simulink model "HANcoder_E407_TTA_CombineModel_Membership_2022a"  (R2023a)
settings: Solver=FixedStepDiscrete  StartTime=0.0  StopTime=1  FixedStep=0.001  RelTol=1e-3
PreLoadFcn:
  | librarySetup
  | eval([bdroot,'_startup']) %Calling [modelName]_startup.m
values from neighbouring files (symbols this model uses):
  ClockOn = Simulink.Parameter    [HANcoder_E407_TTA_Chris_startup.m]    (also in HANcoder_E407_TTA_CombineModel_Membership_2022a_startup.m; HANcoder_E407_TTA_CombineModel_Membership_startup.m; HANcoder_E407_TTA_CombineModel_V2_startup.m; HANcoder_E407_TTA_CombineModel_startup.m)
  controlWidth = Simulink.Parameter    [HANcoder_E407_TTA_CombineModel_Membership_2022a_startup.m]    (also in HANcoder_E407_TTA_CombineModel_Membership_startup.m; HANcoder_E407_TTA_CombineModel_V2_startup.m)
  desiredAngle = Simulink.Parameter    [HANcoder_E407_TTA_CombineModel_Membership_2022a_startup.m]    (also in HANcoder_E407_TTA_CombineModel_Membership_startup.m; HANcoder_E407_TTA_CombineModel_V2_startup.m)
  ErrorBoard1 = Simulink.Parameter    [HANcoder_E407_TTA_CombineModel_Membership_2022a_startup.m]
  ErrorBoard2 = Simulink.Parameter    [HANcoder_E407_TTA_CombineModel_Membership_2022a_startup.m]
  ErrorBoard3 = Simulink.Parameter    [HANcoder_E407_TTA_CombineModel_Membership_2022a_startup.m]
  ErrorBoard4 = Simulink.Parameter    [HANcoder_E407_TTA_CombineModel_Membership_2022a_startup.m]
  ErrorBoard5 = Simulink.Parameter    [HANcoder_E407_TTA_CombineModel_Membership_2022a_startup.m]
  frequency_IRQ = 1000    [HANcoder_E407_TTA_Chris_startup.m]    (also in HANcoder_E407_TTA_CombineModel_Membership_2022a_startup.m; HANcoder_E407_TTA_CombineModel_Membership_startup.m; HANcoder_E407_TTA_CombineModel_V2_startup.m; HANcoder_E407_TTA_CombineModel_startup.m)
  intVal = Simulink.Parameter    [HANcoder_E407_TTA_CombineModel_Membership_2022a_startup.m]    (also in HANcoder_E407_TTA_CombineModel_Membership_startup.m; HANcoder_E407_TTA_CombineModel_V2_startup.m)
  L0b = 1    [HANcoder_E407_KinematicAngleControl_startup.m]    (also in HANcoder_E407_TTA_CombineModel_Membership_2022a_startup.m; HANcoder_E407_TTA_CombineModel_Membership_startup.m; HANcoder_E407_TTA_CombineModel_V2_startup.m; HANcoder_E407_TTA_CombineModel_startup.m)
  L0F = 3    [HANcoder_E407_KinematicAngleControl_startup.m]    (also in HANcoder_E407_TTA_CombineModel_Membership_2022a_startup.m; HANcoder_E407_TTA_CombineModel_Membership_startup.m; HANcoder_E407_TTA_CombineModel_V2_startup.m; HANcoder_E407_TTA_CombineModel_startup.m)
  L1F = 4    [HANcoder_E407_KinematicAngleControl_startup.m]    (also in HANcoder_E407_TTA_CombineModel_Membership_2022a_startup.m; HANcoder_E407_TTA_CombineModel_Membership_startup.m; HANcoder_E407_TTA_CombineModel_V2_startup.m; HANcoder_E407_TTA_CombineModel_startup.m)
  matrixRows = Simulink.Parameter    [HANcoder_E407_TTA_Chris_startup.m]    (also in HANcoder_E407_TTA_CombineModel_Membership_2022a_startup.m; HANcoder_E407_TTA_CombineModel_Membership_startup.m; HANcoder_E407_TTA_CombineModel_V2_startup.m; HANcoder_E407_TTA_CombineModel_startup.m)
  MMBS1_ID = Simulink.Parameter    [HANcoder_E407_TTA_Chris_startup.m]    (also in HANcoder_E407_TTA_CombineModel_Membership_2022a_startup.m; HANcoder_E407_TTA_CombineModel_Membership_startup.m; HANcoder_E407_TTA_CombineModel_V2_startup.m; HANcoder_E407_TTA_CombineModel_startup.m)
  propVal = Simulink.Parameter    [HANcoder_E407_TTA_CombineModel_Membership_2022a_startup.m]    (also in HANcoder_E407_TTA_CombineModel_Membership_startup.m; HANcoder_E407_TTA_CombineModel_V2_startup.m)
  slotTime = Simulink.Parameter    [HANcoder_E407_TTA_Chris_startup.m]    (also in HANcoder_E407_TTA_CombineModel_Membership_2022a_startup.m; HANcoder_E407_TTA_CombineModel_Membership_startup.m; HANcoder_E407_TTA_CombineModel_V2_startup.m; HANcoder_E407_TTA_CombineModel_startup.m)
  SSTM1_ID = Simulink.Parameter    [HANcoder_E407_TTA_Chris_startup.m]    (also in HANcoder_E407_TTA_CombineModel_Membership_2022a_startup.m; HANcoder_E407_TTA_CombineModel_Membership_startup.m; HANcoder_E407_TTA_CombineModel_V2_startup.m; HANcoder_E407_TTA_CombineModel_startup.m)
  SYNC1_ID = Simulink.Parameter    [HANcoder_E407_TTA_Chris_startup.m]    (also in HANcoder_E407_TTA_CombineModel_Membership_2022a_startup.m; HANcoder_E407_TTA_CombineModel_Membership_startup.m; HANcoder_E407_TTA_CombineModel_V2_startup.m; HANcoder_E407_TTA_CombineModel_startup.m)
  TRCK1_ID1 = Simulink.Parameter    [HANcoder_E407_TTA_Chris_startup.m]    (also in HANcoder_E407_TTA_CombineModel_Membership_2022a_startup.m; HANcoder_E407_TTA_CombineModel_Membership_startup.m; HANcoder_E407_TTA_CombineModel_V2_startup.m; HANcoder_E407_TTA_CombineModel_startup.m)
  TRCK1_ID2 = Simulink.Parameter    [HANcoder_E407_TTA_Chris_startup.m]    (also in HANcoder_E407_TTA_CombineModel_Membership_2022a_startup.m; HANcoder_E407_TTA_CombineModel_Membership_startup.m; HANcoder_E407_TTA_CombineModel_V2_startup.m; HANcoder_E407_TTA_CombineModel_startup.m)
  TRCK1_ID3 = Simulink.Parameter    [HANcoder_E407_TTA_Chris_startup.m]    (also in HANcoder_E407_TTA_CombineModel_Membership_2022a_startup.m; HANcoder_E407_TTA_CombineModel_Membership_startup.m; HANcoder_E407_TTA_CombineModel_V2_startup.m; HANcoder_E407_TTA_CombineModel_startup.m)
  TRLS1_ID4 = Simulink.Parameter    [HANcoder_E407_TTA_Chris_startup.m]    (also in HANcoder_E407_TTA_CombineModel_Membership_2022a_startup.m; HANcoder_E407_TTA_CombineModel_Membership_startup.m; HANcoder_E407_TTA_CombineModel_V2_startup.m; HANcoder_E407_TTA_CombineModel_startup.m)
  TRLS1_ID5 = Simulink.Parameter    [HANcoder_E407_TTA_Chris_startup.m]    (also in HANcoder_E407_TTA_CombineModel_Membership_2022a_startup.m; HANcoder_E407_TTA_CombineModel_Membership_startup.m; HANcoder_E407_TTA_CombineModel_V2_startup.m; HANcoder_E407_TTA_CombineModel_startup.m)
undefined symbols (not defined in the file or in its folder): A2, A3, A4, CON2, CON3, CON4, D10, D4, D5
libraries: HANcoder_STM32_Target x23, hdlsllib x12, dspstat3 x2, simulink_extras x2, simulink x1, slpidlib x1, dspswit3 x1
(part 3 of 4)

== system HANcoder_E407_TTA_CombineModel_Membership_2022a/HANcoder STM32 Target - E407-STM32 algorithm/Message selector/SYNC1_TX/CAN send1 ==
  In1 : Inport
  In2 : Inport  Port=2
  In3 : Inport  Port=3
  In4 : Inport  Port=4
  In5 : Inport  Port=5
  In6 : Inport  Port=6
  In7 : Inport  Port=7
  In8 : Inport  Port=8
  In9 : Inport  Port=9
  S-Function : M-S-Function  FunctionName=sfcn_can_send  Parameters=tsamp, canBus, frameType, inputNumber, dataType, byteOrder
  wires:
  In1/1 -> S-Function/1
  In2/1 -> S-Function/2
  In3/1 -> S-Function/3
  In4/1 -> S-Function/4
  In5/1 -> S-Function/5
  In6/1 -> S-Function/6
  In7/1 -> S-Function/7
  In8/1 -> S-Function/8
  In9/1 -> S-Function/9

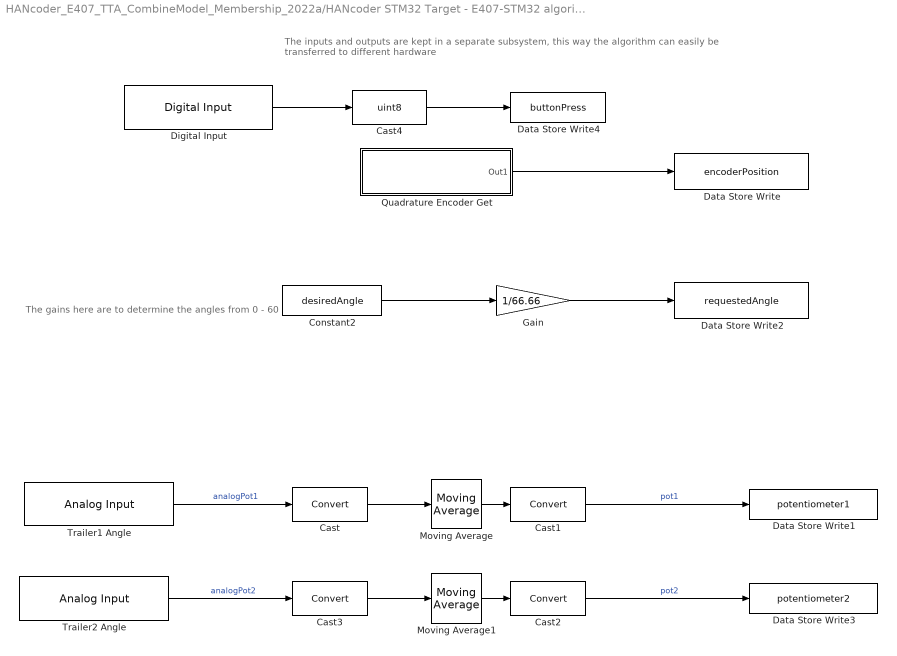
== system HANcoder_E407_TTA_CombineModel_Membership_2022a/HANcoder STM32 Target - E407-STM32 algorithm/Message selector/Slot 5 execution/Inputs ==
  note: The inputs and outputs are kept in a separate subsystem, this way the algorithm can easily be transferred to different hardware
  note: The gains here are to determine the angles from 0 - 60
  Cast{,1..3} (4 alike) : DataTypeConversion  SaturateOnIntegerOverflow=off  RndMeth=Floor
  Cast4 : DataTypeConversion  OutDataTypeStr=uint8  SaturateOnIntegerOverflow=off  RndMeth=Floor
  Constant2 : Constant  Value=desiredAngle
  Data Store Write : DataStoreWrite  DataStoreName=encoderPosition  IndexOptions=Index vector (dialog)  Indices=1  OutputSizes=1
  Data Store Write1 : DataStoreWrite  DataStoreName=potentiometer1  IndexOptions=Index vector (dialog)  Indices=1  OutputSizes=1
  Data Store Write2 : DataStoreWrite  DataStoreName=requestedAngle  IndexOptions=Index vector (dialog)  Indices=1  OutputSizes=1
  Data Store Write3 : DataStoreWrite  DataStoreName=potentiometer2  IndexOptions=Index vector (dialog)  Indices=1  OutputSizes=1
  Data Store Write4 : DataStoreWrite  DataStoreName=buttonPress  IndexOptions=Index vector (dialog)  Indices=1  OutputSizes=1
  Digital Input : HANcoder_STM32_Target/STM32-E407/Digital Inputs/Digital Input  Tag=HANcoder_TARGET_STM32_E407  pinID=WKUP button  config=Pulldown  tsamp=-1
      settings: SourceProductName=HANcoder STM32 Target
  Gain : Gain  Gain=1/66.66  OutDataTypeStr=double  RndMeth=Round
  Moving Average : dspstat3/Moving Average  Method=Sliding window  ForgettingFactorPort=off  SpecifyWindowLength=on  WindowLength=60  OverlapLength=59  AllowArbitraryInputLength=off  ForgettingFactor=0.9  SimulateUsing=Code generation
  Moving Average1 : dspstat3/Moving Average  Method=Sliding window  ForgettingFactorPort=off  SpecifyWindowLength=on  WindowLength=60  OverlapLength=59  AllowArbitraryInputLength=off  ForgettingFactor=0.9  SimulateUsing=Code generation
  Quadrature Encoder Get : Subsystem  Tag=HANcoder_TARGET_STM32_E407  AncestorBlock=HANcoder_STM32_Target/STM32-E407/Timer Inputs/Quadrature Encoder Get  mask(Quadrature Encoder Inputs){moduleID=TIM3: CON4 - D12 & D11 (5V Tolerant), config=Floating, counterReset=off, tsamp=-1}
      mask prompts: moduleID "Quad encoder module"; config "Configuration"; counterReset "Show counter reset input"; tsamp "Sample time"
      mask help:
      | Function
      | ========
      | Reads the counter of the quadrature encoder module.
      |
      | Parameters
      | ==========
      | Quadrature encoder module:
      |   Selects the quadrature encoder module. The channel A and B signals of the
      |   encoder should be connected to the 2 input pins that belong to the module.
      |
      | Configuration:
      |   Determines if the input is floating or is connected to an internal
      |   pull-up or pull-down resistor.
      |
      | Show counter reset input:
      |   Configures if the input port for the counter reset should be shown.
      |
      |
      | Outport
      | ==========
      | 32-bit signed counter. The counter starts at zero and counts up or down
      | depending on the direction of the motor.
      mask init:
      | moduleIDInfoStr = sfcn_quad_encoder_get_mcb(2,moduleID, counterReset, config);
      settings: LibrarySourceBlock=HANcoder_STM32_Target/STM32-E407/Timer Inputs/Quadrature Encoder Get  CopyFcn=sfcn_quad_encoder_get_chk();  MoveFcn=drawLogos
      mask Help: web('sfcn_quad_encoder_get.html');
      mask TypeOptions moduleID: TIM1: CON PE - 12 & 14 (5V Tolerant) | TIM3: CON4 - D12 & D11 (5V Tolerant) | TIM4: CON PD - 15 & 16 (5V Tolerant) | TIM8: UEXT - 3 & 4 (5V Tolerant)
      mask Callback moduleID: sfcn_quad_encoder_get_chk();
      mask TypeOptions config: Floating | Pullup | Pulldown
      mask Display: fprintf('Quad Encoder Get\n%s', moduleIDInfoStr);patch([135 141 141],[8 14 2],[1 0 0]);patch([143 143 149],[14 2 8],[0 0 0.35]);
  Trailer1 Angle : HANcoder_STM32_Target/STM32-E407/Analog Inputs/Analog Input  Tag=HANcoder_TARGET_STM32_E407  pinID=CON2 - A2  tsamp=-1  filtered=off
      settings: SourceProductName=HANcoder STM32 Target
  Trailer2 Angle : HANcoder_STM32_Target/STM32-E407/Analog Inputs/Analog Input  Tag=HANcoder_TARGET_STM32_E407  pinID=CON2 - A3  tsamp=-1  filtered=off
      settings: SourceProductName=HANcoder STM32 Target
  wires:
  Constant2/1 -> Gain/1
  Gain/1 -> Data Store Write2/1
  Quadrature Encoder Get/1(Out1) -> Data Store Write/1
  Trailer1 Angle/1 -> Cast/1  "analogPot1"
  Trailer2 Angle/1 -> Cast3/1  "analogPot2"
  Moving Average/1 -> Cast1/1
  Moving Average1/1 -> Cast2/1
  Cast/1 -> Moving Average/1
  Cast1/1 -> Data Store Write1/1  "pot1"
  Cast2/1 -> Data Store Write3/1  "pot2"
  Cast3/1 -> Moving Average1/1
  Digital Input/1 -> Cast4/1
  Cast4/1 -> Data Store Write4/1

== system HANcoder_E407_TTA_CombineModel_Membership_2022a/HANcoder STM32 Target - E407-STM32 algorithm/Message selector/Slot 5 execution/Outputs ==
  note: The inputs and outputs are kept in a separate subsystem, this way the algorithm can easily be transferred to different hardware
  PWM mospeed : Inport
  CW signal : Inport  Port=2
  CCW signal : Inport  Port=3
  Node : Inport  Port=4
  Data Store Read : DataStoreRead  DataStoreName=Master_ID  IndexOptions=Index vector (dialog)  Indices=1  OutputSizes=1
  Digital Output : HANcoder_STM32_Target/STM32-E407/Digital Outputs/Digital Output  Tag=HANcoder_TARGET_STM32_E407  pinID=CON3 - D4  config=Push pull  tsamp=-1
      settings: SourceProductName=HANcoder STM32 Target
  Digital Output1 : HANcoder_STM32_Target/STM32-E407/Digital Outputs/Digital Output  Tag=HANcoder_TARGET_STM32_E407  pinID=CON3 - D5  config=Push pull  tsamp=-1
      settings: SourceProductName=HANcoder STM32 Target
  Digital Output2 : HANcoder_STM32_Target/STM32-E407/Digital Outputs/Digital Output  Tag=HANcoder_TARGET_STM32_E407  pinID=LED  config=Push pull  tsamp=-1
      settings: SourceProductName=HANcoder STM32 Target
  Equal : RelationalOperator  Operator===  OutDataTypeStr=boolean  RndMeth=Simplest  InputSameDT=off
  PWM Duty Cycle : HANcoder_STM32_Target/STM32-E407/PWM Outputs/PWM Duty Cycle  Tag=HANcoder_TARGET_STM32_E407  pinID=CON2 - A4  tsamp=-1
      settings: SourceProductName=HANcoder STM32 Target
  PWM Init : Subsystem  Tag=HANcoder_TARGET_STM32_E407  AncestorBlock=HANcoder_STM32_Target/STM32-E407/PWM Outputs/PWM Init  mask(Pulse Width Modulation Initialization){moduleID=TIM14: A4 & n/a & n/a & n/a, frequency=10253, alignment=Edge aligned, enableIRQoutput=off, ch1On=on, ch1Pol=Active high, ch1Inv=off, ch2On=on, ch2Pol=Active high, ch2Inv=off, ch3On=off, ch3Pol=Active high, ch3Inv=off, ch4On=off, ch4Pol=Active high, ch4Inv=off}
      mask prompts: moduleID "PWM module"; frequency "Signal frequency [Hz]"; alignment "Signal alignment"; enableIRQoutput "Enable IRQ output"; ch1On "Generate PWM signal on channel 1"; ch1Pol "Select signal polarity"; ch1Inv "Enable inverted signal on additional output pin"; ch2On "Generate PWM signal on channel 2"; ch2Pol "Select signal polarity"; ch2Inv "Enable inverted signal on additional output pin"; ch3On "Generate PWM signal on channel 3"; ch3Pol "Select signal polarity"; ch3Inv "Enable inverted signal on additional output pin"; ch4On "Generate PWM signal on channel 4"; ch4Pol "Select signal polarity"; ch4Inv "Enable inverted signal on additional output pin"
      mask help:
      | Function
      | ========
      | A 'PWM Init' block configures one of the STM32 timer modules for PWM
      | functionality, allowing a PWM signal to be generated on up to 4 timer
      | channels and their associated output pins.
      |
      | Parameters
      | ==========
      | General - PWM module:
      |   Select the PWM module to use. The name in the combo box contains
      |   information about which pins on the target belong to this timer module.
      |   Also the first pin corresponds with the first channel and so on:
      |   TIMx: Ch1 & Ch2 & Ch3...
      |
      | General - Signal frequency:
      |   Determines the signal frequency in Hz. If you click 'Apply' after entering
      |   the desired frequency it will automatically be adjusted to the closest
      |   supported value.
      |
      | General - Signal Aligment:
      |   Determines the aligment of the signal. It can either be edge aligned or
      |   center aligned.
      |
      | General - Enable IRQ output
      |   Controls whether or not the IRQ output is available.
      |
      | Channel x - Generate PWM signal on channel x:
      |   Enable to configure the channel for PWM functionality so that the PWM signal
      |   is outputted on the channel's associated microcontroller pin.
      |
      | Channel x - Signal polarity:
      |   Selects the polarity of the signal.
      |
      | Channel x - Enable inverted signal on additional output pin:
      |   When enabled, a second PWM signal will be generated on an additional
      |   microcontroller pin where the signal is an exact inversion of the first signal.
      mask init:
      | moduleIDInfoStr = sfcn_pwmout_init_mcb(2, moduleID, frequency, alignment, enableIRQoutput, ch1On, ch2On, ch3On, ch4On, ch1Pol, ch2Pol, ch3Pol, ch4Pol, ch1Inv, ch2Inv, ch3Inv, ch4Inv);
      settings: LibrarySourceBlock=HANcoder_STM32_Target/STM32-E407/PWM Outputs/PWM Init  CopyFcn=sfcn_pwmout_init_chk();  MoveFcn=drawLogos
      mask Help: web('sfcn_pwmout_init.html');
      mask TypeOptions moduleID: TIM1:   PE12 & PE14 & PE16 & PE17 + N-channels PE11 & PE13 & PE15 | TIM2:   D13 & n/a & n/a & n/a | TIM3:   D12 & D11 & n/a & n/a | TIM4:   PD15 & PD16 &n/a & n/a | TIM8:   UEXT3 & UEXT4 & n/a & n/a | TIM9:   D4 & D5 & n/a & n/a | TIM10: A1 & n/a & n/a & n/a | TIM11: A2 & n/a & n/a & n/a | TIM13: A3 & n/a & n/a & n/a | TIM14: A4 & n/a & n/a & n/a
      mask Callback moduleID: sfcn_pwmout_init_chk();
      mask TypeOptions alignment: Edge aligned | Center aligned
      mask TypeOptions ch1Pol: Active high | Active low
      mask TypeOptions ch2Pol: Active high | Active low
      mask TypeOptions ch3Pol: Active high | Active low
      mask TypeOptions ch4Pol: Active high | Active low
      mask Display: fprintf('PWM Init\n%s', moduleIDInfoStr);patch([195 201 201],[8 14 2],[1 0 0]);patch([203 203 209],[14 2 8],[0 0 0.35]);
  wires:
  CCW signal/1 -> Digital Output1/1
  CW signal/1 -> Digital Output/1
  PWM mospeed/1 -> PWM Duty Cycle/1
  Node/1 -> Equal/1
  Equal/1 -> Digital Output2/1
  Data Store Read/1 -> Equal/2

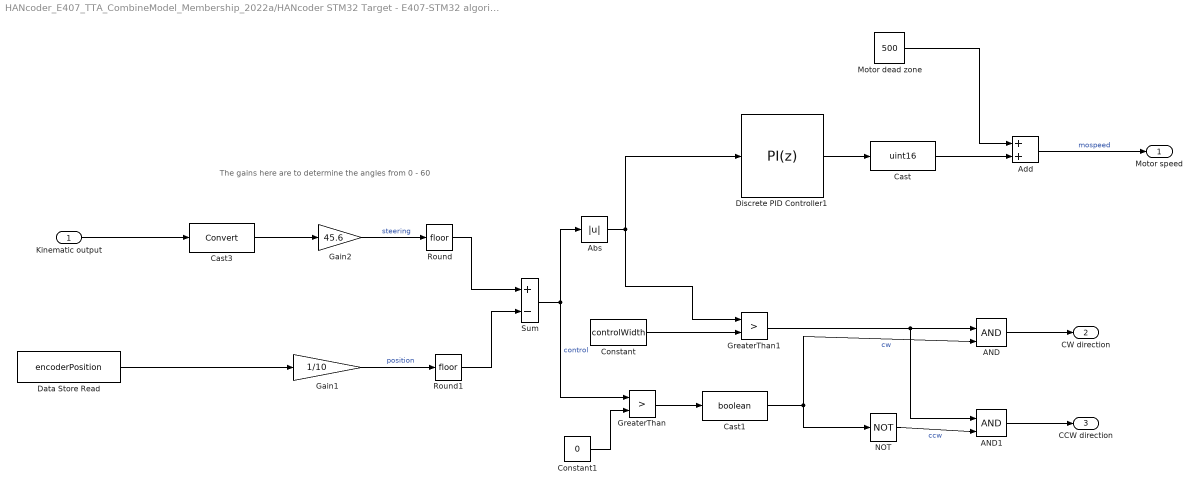
== system HANcoder_E407_TTA_CombineModel_Membership_2022a/HANcoder STM32 Target - E407-STM32 algorithm/Message selector/Subsystem/Control Algorithm ==
  note: The gains here are to determine the angles from 0 - 60
  Kinematic output : Inport
  AND : Logic  IconShape=distinctive  AllPortsSameDT=off  OutDataTypeStr=boolean
  AND1 : Logic  IconShape=distinctive  AllPortsSameDT=off  OutDataTypeStr=boolean
  Abs : Abs  OutDataTypeStr=double  SaturateOnIntegerOverflow=off
  Add : Sum  AccumDataTypeStr=uint16
  Cast : DataTypeConversion  OutDataTypeStr=uint16  SaturateOnIntegerOverflow=off  RndMeth=Floor
  Cast1 : DataTypeConversion  OutDataTypeStr=boolean  SaturateOnIntegerOverflow=off  RndMeth=Floor
  Cast3 : DataTypeConversion  SaturateOnIntegerOverflow=off  RndMeth=Floor
  Constant : Constant  Value=controlWidth
  Constant1 : Constant  Value=0
  Data Store Read : DataStoreRead  DataStoreName=encoderPosition  IndexOptions=Index vector (dialog)  Indices=1  OutputSizes=1
  Discrete PID Controller1 : slpidlib/PID Controller  Controller=PI  Form=Parallel  TimeDomain=Discrete-time  UseExternalTs=off  SampleTime=-1  IntegratorMethod=Forward Euler  FilterMethod=Forward Euler  ControllerParametersSource=internal  P=propVal  I=intVal  UseKiTs=on  D=0.5  N=100  UseFilter=on  TunerSelectOption=Transfer Function Based (PID Tuner App)  InitialConditionSource=internal  InitialConditionForIntegrator=0  InitialConditionForFilter=0  DifferentiatorICPrevScaledInput=0  ExternalReset=none  TrackingMode=off  Kt=1  LimitOutput=on  SatLimitsSource=internal  UpperSaturationLimit=300  LowerSaturationLimit=0  LinearizeAsGain=off  AntiWindupMode=clamping  Kb=1  LimitIntegrator=off  UpperIntegratorSaturationLimit=inf  LowerIntegratorSaturationLimit=-inf  POutMin=[]  POutMax=[]  IOutMin=[]  IOutMax=[]  DOutMin=[]  DOutMax=[]  NOutMin=[]  NOutMax=[]  SumOutMin=[]  SumOutMax=[]  SaturationOutMin=[]  SaturationOutMax=[]  PParamMin=[]  PParamMax=[]  IParamMin=[]  IParamMax=[]  DParamMin=[]  DParamMax=[]  NParamMin=[]  NParamMax=[]  KbParamMin=[]  KbParamMax=[]  KtParamMin=[]  KtParamMax=[]  KbOutMin=[]  KbOutMax=[]  KtOutMin=[]  KtOutMax=[]  IntegratorOutMin=[]  IntegratorOutMax=[]  FilterOutMin=[]  FilterOutMax=[]  SumI1OutMin=[]  SumI1OutMax=[]  SumI2OutMin=[]  SumI2OutMax=[]  SumI3OutMin=[]  SumI3OutMax=[]  SumI4OutMin=[]  SumI4OutMax=[]  SumDOutMin=[]  SumDOutMax=[]  DifferentiatorOutMin=[]  DifferentiatorOutMax=[]  FilterDiffOutCoefMin=[]  FilterDiffOutCoefMax=[]  ReciprocalOutMin=[]  ReciprocalOutMax=[]  SumDenOutMin=[]  SumDenOutMax=[]  SumNumOutMin=[]  SumNumOutMax=[]  DivideOutMin=[]  DivideOutMax=[]  UdiffTsProdOutMin=[]  UdiffTsProdOutMax=[]  NTsProdOutMin=[]  NTsProdOutMax=[]  UintegralTsProdOutMin=[]  UintegralTsProdOutMax=[]  UngainTsProdOutMin=[]  UngainTsProdOutMax=[]  ClampingZeroOutDataTypeStr=Inherit: Inherit via back propagation  ClampingZeroOutMin=[]  ClampingZeroOutMax=[]  FilterDenConstantOutDataTypeStr=Inherit: Inherit via back propagation  FilterDenConstantOutMin=[]  FilterDenConstantOutMax=[]  PCopyOutDataTypeStr=Inherit: Inherit via back propagation  PCopyOutMin=[]  PCopyOutMax=[]  NCopyOutDataTypeStr=Inherit: Inherit via back propagation  NCopyOutMin=[]  NCopyOutMax=[]  IntegratorContinuousStateAttributes=''  IntegratorStateMustResolveToSignalObject=off  IntegratorRTWStateStorageClass=Auto  FilterContinuousStateAttributes=''  FilterStateMustResolveToSignalObject=off  FilterRTWStateStorageClass=Auto  ParallelPVariant=InternalParameters  IdealPVariant=Disabled  IVariant=InternalParameters  DVariant=Disabled  IntegratorVariant=Discrete  SatVariant=Enabled  AWVariant=DiscClampingParallel  PCopyVariant=Disabled  TRVariant=Disabled  FdbkBlocksVariant=Forward  IdealPFdbkVariant=Disabled  SatFdbkVariant=Disabled  DerivativeFilterVariant=Disabled  NVariant=Disabled  NCopyVariant=Disabled_SignalSpec  FilterICVariant=Disabled  IntegratorICVariant=InternalICs  ExternalResetVariant=Disabled  TRSumVariant=Passthrough  SumFdbkVariant=Disabled  SumVariant=Sum_PI  TsampFilterVariant=InternalTs  TsampNgainVariant=Passthrough  TsampIntegralVariant=Disabled_SignalSpec  ExternalSaturationOutDataTypeStr=Inherit: Same as second input
  Gain1 : Gain  Gain=1/10  OutDataTypeStr=double
  Gain2 : Gain  Gain=45.6
  GreaterThan : RelationalOperator  Operator=>  OutDataTypeStr=boolean  RndMeth=Simplest  InputSameDT=off
  GreaterThan1 : RelationalOperator  Operator=>  OutDataTypeStr=boolean  RndMeth=Simplest  InputSameDT=off
  Motor dead zone : Constant  Value=500  OutDataTypeStr=uint16
  NOT : Logic  Operator=NOT  IconShape=distinctive  AllPortsSameDT=off  OutDataTypeStr=boolean
  Round : Rounding
  Round1 : Rounding
  Sum : Sum  Inputs=+-
  Motor speed : Outport
  CW direction : Outport  Port=2
  CCW direction : Outport  Port=3
  wires:
  Motor dead zone/1 -> Add/1
  Sum/1 -> GreaterThan/1, Abs/1  "control"
  Abs/1 -> Discrete PID Controller1/1, GreaterThan1/1
  GreaterThan/1 -> Cast1/1
  Cast1/1 -> AND/2, NOT/1  "cw"
  Add/1 -> Motor speed/1  "mospeed"
  Constant1/1 -> GreaterThan/2
  Gain1/1 -> Round1/1  "position"
  Discrete PID Controller1/1 -> Cast/1
  Gain2/1 -> Round/1  "steering"
  Kinematic output/1 -> Cast3/1
  Round/1 -> Sum/1
  Round1/1 -> Sum/2
  Data Store Read/1 -> Gain1/1
  Cast3/1 -> Gain2/1
  Cast/1 -> Add/2
  GreaterThan1/1 -> AND/1, AND1/1
  Constant/1 -> GreaterThan1/2
  AND/1 -> CW direction/1
  NOT/1 -> AND1/2  "ccw"
  AND1/1 -> CCW direction/1

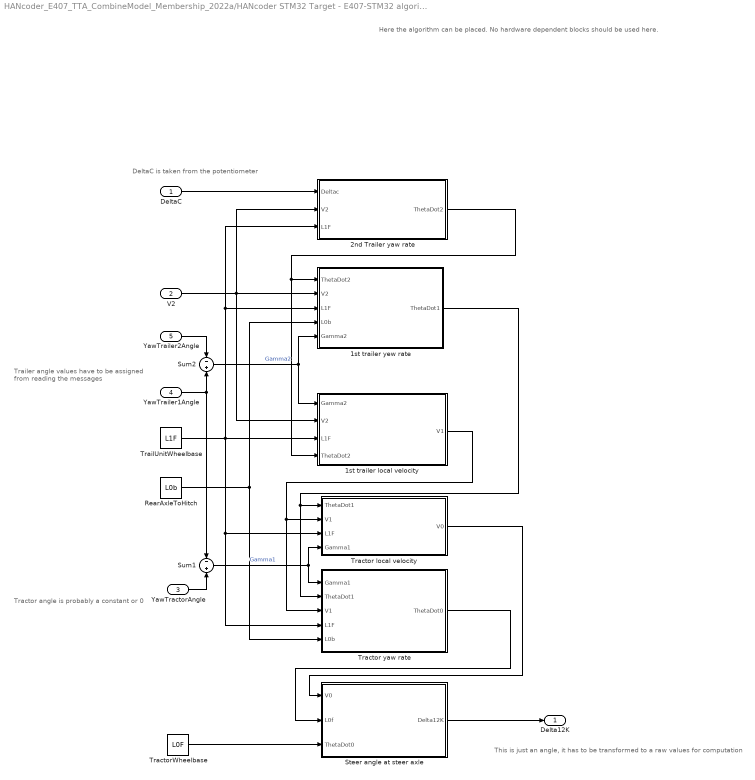
== system HANcoder_E407_TTA_CombineModel_Membership_2022a/HANcoder STM32 Target - E407-STM32 algorithm/Message selector/Subsystem/Kinematic Algorithm ==
  note: Here the algorithm can be placed. No hardware dependent blocks should be used here.
  note: Tractor angle is probably a constant or 0
  note: DeltaC is taken from the potentiometer
  note: This is just an angle, it has to be transformed to a raw values for computation
  note: Trailer angle values have to be assigned
      |  from reading the messages
  DeltaC : Inport
  V2 : Inport  Port=2
  YawTractorAngle : Inport  Port=3
  YawTrailer1Angle : Inport  Port=4
  YawTrailer2Angle : Inport  Port=5
  1st trailer local velocity : Subsystem
  1st trailer yew rate : Subsystem
  2nd Trailer yaw rate : Subsystem
  RearAxleToHitch : Constant  Value=L0b
  Steer angle at steer axle : Subsystem
  Sum1 : Sum  Inputs=-+
  Sum2 : Sum  Inputs=-+
  Tractor local velocity : Subsystem
  Tractor yaw rate : Subsystem
  TractorWheelbase : Constant  Value=L0F
  TrailUnitWheelbase : Constant  Value=L1F
  Delta12K : Outport
  wires:
  Tractor local velocity/1(V0) -> Steer angle at steer axle/1(V0)
  RearAxleToHitch/1 -> Tractor yaw rate/5(L0b), 1st trailer yew rate/4(L0b)
  2nd Trailer yaw rate/1(ThetaDot2) -> 1st trailer local velocity/4(ThetaDot2), 1st trailer yew rate/1(ThetaDot2)
  Sum2/1 -> 1st trailer local velocity/1(Gamma2), 1st trailer yew rate/5(Gamma2)  "Gamma2"
  Sum1/1 -> Tractor yaw rate/1(Gamma1), Tractor local velocity/4(Gamma1)  "Gamma1"
  1st trailer yew rate/1(ThetaDot1) -> Tractor yaw rate/2(ThetaDot1), Tractor local velocity/1(ThetaDot1)
  YawTrailer1Angle/1 -> Sum1/1, Sum2/2
  V2/1 -> 1st trailer yew rate/2(V2), 1st trailer local velocity/2(V2), 2nd Trailer yaw rate/2(V2)
  YawTrailer2Angle/1 -> Sum2/1
  TrailUnitWheelbase/1 -> Tractor yaw rate/4(L1F), Tractor local velocity/3(L1F), 1st trailer local velocity/3(L1F), 1st trailer yew rate/3(L1F), 2nd Trailer yaw rate/3(L1F)
  Steer angle at steer axle/1(Delta12K) -> Delta12K/1
  1st trailer local velocity/1(V1) -> Tractor yaw rate/3(V1), Tractor local velocity/2(V1)
  DeltaC/1 -> 2nd Trailer yaw rate/1(Deltac)
  Tractor yaw rate/1(ThetaDot0) -> Steer angle at steer axle/2(L0f)
  TractorWheelbase/1 -> Steer angle at steer axle/3(ThetaDot0)
  YawTractorAngle/1 -> Sum1/2

== system HANcoder_E407_TTA_CombineModel_Membership_2022a/HANcoder STM32 Target - E407-STM32 algorithm/Message selector/TRCK1_ID2_RX/CAN receive1 ==
  In1 : Inport
  Enabled Subsystem : Subsystem  TreatAsAtomicUnit=on
  S-Function : M-S-Function  FunctionName=sfcn_can_receive  Parameters=tsamp, canBus, outputNumber, dataType, byteOrder
  Out1 : Outport
  Out2 : Outport  Port=2
  Out3 : Outport  Port=3
  Out4 : Outport  Port=4
  Out5 : Outport  Port=5
  Out6 : Outport  Port=6
  Out7 : Outport  Port=7
  Out8 : Outport  Port=8
  Out9 : Outport  Port=9
  wires:
  S-Function/9 -> Enabled Subsystem/8(In8)
  S-Function/4 -> Enabled Subsystem/3(In3)
  S-Function/5 -> Enabled Subsystem/4(In4)
  S-Function/8 -> Enabled Subsystem/7(In7)
  S-Function/7 -> Enabled Subsystem/6(In6)
  S-Function/6 -> Enabled Subsystem/5(In5)
  Enabled Subsystem/8(Out8) -> Out9/1
  Enabled Subsystem/7(Out7) -> Out8/1
  Enabled Subsystem/6(Out6) -> Out7/1
  Enabled Subsystem/5(Out5) -> Out6/1
  Enabled Subsystem/4(Out4) -> Out5/1
  Enabled Subsystem/3(Out3) -> Out4/1
  Enabled Subsystem/2(Out2) -> Out3/1
  Enabled Subsystem/1(Out1) -> Out2/1
  S-Function/3 -> Enabled Subsystem/2(In2)
  S-Function/2 -> Enabled Subsystem/1(In1)
  S-Function/1 -> Out1/1, Enabled Subsystem/Enable
  In1/1 -> S-Function/1

== system HANcoder_E407_TTA_CombineModel_Membership_2022a/HANcoder STM32 Target - E407-STM32 algorithm/Message selector/TRCK1_ID2_TX/CAN send1 ==
  In1 : Inport
  In2 : Inport  Port=2
  In3 : Inport  Port=3
  In4 : Inport  Port=4
  In5 : Inport  Port=5
  In6 : Inport  Port=6
  Gnd7 : Ground
  Gnd8 : Ground
  Gnd9 : Ground
  S-Function : M-S-Function  FunctionName=sfcn_can_send  Parameters=tsamp, canBus, frameType, inputNumber, dataType, byteOrder
  wires:
  In1/1 -> S-Function/1
  In2/1 -> S-Function/2
  In3/1 -> S-Function/3
  In4/1 -> S-Function/4
  In5/1 -> S-Function/5
  In6/1 -> S-Function/6
  Gnd7/1 -> S-Function/7
  Gnd8/1 -> S-Function/8
  Gnd9/1 -> S-Function/9

== system HANcoder_E407_TTA_CombineModel_Membership_2022a/HANcoder STM32 Target - E407-STM32 algorithm/Message selector/TRCK1_ID2_TX/uint16to2uint1 ==
  input : Inport
  Bit Shift : hdlsllib/Logic and Bit Operations/Bit Shift  mode=Shift Right Logical  N=8
  Cast : DataTypeConversion  OutDataTypeStr=uint8  SaturateOnIntegerOverflow=off  RndMeth=Floor
  Cast1 : DataTypeConversion  OutDataTypeStr=uint8  SaturateOnIntegerOverflow=off  RndMeth=Floor
  msb : Outport
  lsb : Outport  Port=2
  wires:
  Bit Shift/1 -> Cast/1
  input/1 -> Cast1/1, Bit Shift/1
  Cast/1 -> msb/1
  Cast1/1 -> lsb/1

== system HANcoder_E407_TTA_CombineModel_Membership_2022a/HANcoder STM32 Target - E407-STM32 algorithm/Message selector/TRCK1_ID2_TX/uint16to2uint8 ==
  input : Inport
  Bit Shift : hdlsllib/Logic and Bit Operations/Bit Shift  mode=Shift Right Logical  N=8
  Cast : DataTypeConversion  OutDataTypeStr=uint8  SaturateOnIntegerOverflow=off  RndMeth=Floor
  Cast1 : DataTypeConversion  OutDataTypeStr=uint8  SaturateOnIntegerOverflow=off  RndMeth=Floor
  msb : Outport
  lsb : Outport  Port=2
  wires:
  Bit Shift/1 -> Cast/1
  input/1 -> Cast1/1, Bit Shift/1
  Cast/1 -> msb/1
  Cast1/1 -> lsb/1

== system HANcoder_E407_TTA_CombineModel_Membership_2022a/HANcoder STM32 Target - E407-STM32 algorithm/Message selector/TRCK1_ID3_TX/CAN send1 ==
  In1 : Inport
  In2 : Inport  Port=2
  In3 : Inport  Port=3
  In4 : Inport  Port=4
  In5 : Inport  Port=5
  In6 : Inport  Port=6
  Gnd7 : Ground
  Gnd8 : Ground
  Gnd9 : Ground
  S-Function : M-S-Function  FunctionName=sfcn_can_send  Parameters=tsamp, canBus, frameType, inputNumber, dataType, byteOrder
  wires:
  In1/1 -> S-Function/1
  In2/1 -> S-Function/2
  In3/1 -> S-Function/3
  In4/1 -> S-Function/4
  In5/1 -> S-Function/5
  In6/1 -> S-Function/6
  Gnd7/1 -> S-Function/7
  Gnd8/1 -> S-Function/8
  Gnd9/1 -> S-Function/9

== system HANcoder_E407_TTA_CombineModel_Membership_2022a/HANcoder STM32 Target - E407-STM32 algorithm/Message selector/TRCK1_ID3_TX/uint16to2uint1 ==
  input : Inport
  Bit Shift : hdlsllib/Logic and Bit Operations/Bit Shift  mode=Shift Right Logical  N=8
  Cast : DataTypeConversion  OutDataTypeStr=uint8  SaturateOnIntegerOverflow=off  RndMeth=Floor
  Cast1 : DataTypeConversion  OutDataTypeStr=uint8  SaturateOnIntegerOverflow=off  RndMeth=Floor
  msb : Outport
  lsb : Outport  Port=2
  wires:
  Bit Shift/1 -> Cast/1
  input/1 -> Cast1/1, Bit Shift/1
  Cast/1 -> msb/1
  Cast1/1 -> lsb/1

== system HANcoder_E407_TTA_CombineModel_Membership_2022a/HANcoder STM32 Target - E407-STM32 algorithm/Message selector/TRCK1_ID3_TX/uint16to2uint8 ==
  input : Inport
  Bit Shift : hdlsllib/Logic and Bit Operations/Bit Shift  mode=Shift Right Logical  N=8
  Cast : DataTypeConversion  OutDataTypeStr=uint8  SaturateOnIntegerOverflow=off  RndMeth=Floor
  Cast1 : DataTypeConversion  OutDataTypeStr=uint8  SaturateOnIntegerOverflow=off  RndMeth=Floor
  msb : Outport
  lsb : Outport  Port=2
  wires:
  Bit Shift/1 -> Cast/1
  input/1 -> Cast1/1, Bit Shift/1
  Cast/1 -> msb/1
  Cast1/1 -> lsb/1

== system HANcoder_E407_TTA_CombineModel_Membership_2022a/HANcoder STM32 Target - E407-STM32 algorithm/Message selector/TRCK1_RX/CAN receive1 ==
  In1 : Inport
  Enabled Subsystem : Subsystem  TreatAsAtomicUnit=on
  S-Function : M-S-Function  FunctionName=sfcn_can_receive  Parameters=tsamp, canBus, outputNumber, dataType, byteOrder
  Out1 : Outport
  Out2 : Outport  Port=2
  Out3 : Outport  Port=3
  Out4 : Outport  Port=4
  Out5 : Outport  Port=5
  Out6 : Outport  Port=6
  Out7 : Outport  Port=7
  Out8 : Outport  Port=8
  Out9 : Outport  Port=9
  wires:
  S-Function/9 -> Enabled Subsystem/8(In8)
  S-Function/4 -> Enabled Subsystem/3(In3)
  S-Function/5 -> Enabled Subsystem/4(In4)
  S-Function/8 -> Enabled Subsystem/7(In7)
  S-Function/7 -> Enabled Subsystem/6(In6)
  S-Function/6 -> Enabled Subsystem/5(In5)
  Enabled Subsystem/8(Out8) -> Out9/1
  Enabled Subsystem/7(Out7) -> Out8/1
  Enabled Subsystem/6(Out6) -> Out7/1
  Enabled Subsystem/5(Out5) -> Out6/1
  Enabled Subsystem/4(Out4) -> Out5/1
  Enabled Subsystem/3(Out3) -> Out4/1
  Enabled Subsystem/2(Out2) -> Out3/1
  Enabled Subsystem/1(Out1) -> Out2/1
  S-Function/3 -> Enabled Subsystem/2(In2)
  S-Function/2 -> Enabled Subsystem/1(In1)
  S-Function/1 -> Out1/1, Enabled Subsystem/Enable
  In1/1 -> S-Function/1

== system HANcoder_E407_TTA_CombineModel_Membership_2022a/HANcoder STM32 Target - E407-STM32 algorithm/Message selector/TRCK1_TX/CAN send1 ==
  In1 : Inport
  In2 : Inport  Port=2
  In3 : Inport  Port=3
  In4 : Inport  Port=4
  In5 : Inport  Port=5
  In6 : Inport  Port=6
  Gnd7 : Ground
  Gnd8 : Ground
  Gnd9 : Ground
  S-Function : M-S-Function  FunctionName=sfcn_can_send  Parameters=tsamp, canBus, frameType, inputNumber, dataType, byteOrder
  wires:
  In1/1 -> S-Function/1
  In2/1 -> S-Function/2
  In3/1 -> S-Function/3
  In4/1 -> S-Function/4
  In5/1 -> S-Function/5
  In6/1 -> S-Function/6
  Gnd7/1 -> S-Function/7
  Gnd8/1 -> S-Function/8
  Gnd9/1 -> S-Function/9

== system HANcoder_E407_TTA_CombineModel_Membership_2022a/HANcoder STM32 Target - E407-STM32 algorithm/Message selector/TRCK1_TX/uint16to2uint1 ==
  input : Inport
  Bit Shift : hdlsllib/Logic and Bit Operations/Bit Shift  mode=Shift Right Logical  N=8
  Cast : DataTypeConversion  OutDataTypeStr=uint8  SaturateOnIntegerOverflow=off  RndMeth=Floor
  Cast1 : DataTypeConversion  OutDataTypeStr=uint8  SaturateOnIntegerOverflow=off  RndMeth=Floor
  msb : Outport
  lsb : Outport  Port=2
  wires:
  Bit Shift/1 -> Cast/1
  input/1 -> Cast1/1, Bit Shift/1
  Cast/1 -> msb/1
  Cast1/1 -> lsb/1

== system HANcoder_E407_TTA_CombineModel_Membership_2022a/HANcoder STM32 Target - E407-STM32 algorithm/Message selector/TRCK1_TX/uint16to2uint8 ==
  input : Inport
  Bit Shift : hdlsllib/Logic and Bit Operations/Bit Shift  mode=Shift Right Logical  N=8
  Cast : DataTypeConversion  OutDataTypeStr=uint8  SaturateOnIntegerOverflow=off  RndMeth=Floor
  Cast1 : DataTypeConversion  OutDataTypeStr=uint8  SaturateOnIntegerOverflow=off  RndMeth=Floor
  msb : Outport
  lsb : Outport  Port=2
  wires:
  Bit Shift/1 -> Cast/1
  input/1 -> Cast1/1, Bit Shift/1
  Cast/1 -> msb/1
  Cast1/1 -> lsb/1

== system HANcoder_E407_TTA_CombineModel_Membership_2022a/HANcoder STM32 Target - E407-STM32 algorithm/Message selector/TRCK_ID3_RX/CAN receive1 ==
  In1 : Inport
  Enabled Subsystem : Subsystem  TreatAsAtomicUnit=on
  S-Function : M-S-Function  FunctionName=sfcn_can_receive  Parameters=tsamp, canBus, outputNumber, dataType, byteOrder
  Out1 : Outport
  Out2 : Outport  Port=2
  Out3 : Outport  Port=3
  Out4 : Outport  Port=4
  Out5 : Outport  Port=5
  Out6 : Outport  Port=6
  Out7 : Outport  Port=7
  Out8 : Outport  Port=8
  Out9 : Outport  Port=9
  wires:
  S-Function/9 -> Enabled Subsystem/8(In8)
  S-Function/4 -> Enabled Subsystem/3(In3)
  S-Function/5 -> Enabled Subsystem/4(In4)
  S-Function/8 -> Enabled Subsystem/7(In7)
  S-Function/7 -> Enabled Subsystem/6(In6)
  S-Function/6 -> Enabled Subsystem/5(In5)
  Enabled Subsystem/8(Out8) -> Out9/1
  Enabled Subsystem/7(Out7) -> Out8/1
  Enabled Subsystem/6(Out6) -> Out7/1
  Enabled Subsystem/5(Out5) -> Out6/1
  Enabled Subsystem/4(Out4) -> Out5/1
  Enabled Subsystem/3(Out3) -> Out4/1
  Enabled Subsystem/2(Out2) -> Out3/1
  Enabled Subsystem/1(Out1) -> Out2/1
  S-Function/3 -> Enabled Subsystem/2(In2)
  S-Function/2 -> Enabled Subsystem/1(In1)
  S-Function/1 -> Out1/1, Enabled Subsystem/Enable
  In1/1 -> S-Function/1

== system HANcoder_E407_TTA_CombineModel_Membership_2022a/HANcoder STM32 Target - E407-STM32 algorithm/Message selector/TRLS_ID4_RX/2bytes2uint16 ==
  MSB : Inport
  LSB : Inport  Port=2
  Add : Sum
  Bit Shift : hdlsllib/Logic and Bit Operations/Bit Shift  mode=Shift Left Logical  N=8
  Cast : DataTypeConversion  OutDataTypeStr=uint16  SaturateOnIntegerOverflow=off  RndMeth=Floor
  Cast1 : DataTypeConversion  OutDataTypeStr=uint16  SaturateOnIntegerOverflow=off  RndMeth=Floor
  uint16Out : Outport
  wires:
  Cast/1 -> Bit Shift/1
  Bit Shift/1 -> Add/1
  Cast1/1 -> Add/2
  LSB/1 -> Cast1/1
  MSB/1 -> Cast/1
  Add/1 -> uint16Out/1

== system HANcoder_E407_TTA_CombineModel_Membership_2022a/HANcoder STM32 Target - E407-STM32 algorithm/Message selector/TRLS_ID4_RX/CAN receive1 ==
  In1 : Inport
  Enabled Subsystem : Subsystem  TreatAsAtomicUnit=on
  S-Function : M-S-Function  FunctionName=sfcn_can_receive  Parameters=tsamp, canBus, outputNumber, dataType, byteOrder
  Out1 : Outport
  Out2 : Outport  Port=2
  Out3 : Outport  Port=3
  Out4 : Outport  Port=4
  Out5 : Outport  Port=5
  Out6 : Outport  Port=6
  Out7 : Outport  Port=7
  Out8 : Outport  Port=8
  Out9 : Outport  Port=9
  wires:
  S-Function/9 -> Enabled Subsystem/8(In8)
  S-Function/4 -> Enabled Subsystem/3(In3)
  S-Function/5 -> Enabled Subsystem/4(In4)
  S-Function/8 -> Enabled Subsystem/7(In7)
  S-Function/7 -> Enabled Subsystem/6(In6)
  S-Function/6 -> Enabled Subsystem/5(In5)
  Enabled Subsystem/8(Out8) -> Out9/1
  Enabled Subsystem/7(Out7) -> Out8/1
  Enabled Subsystem/6(Out6) -> Out7/1
  Enabled Subsystem/5(Out5) -> Out6/1
  Enabled Subsystem/4(Out4) -> Out5/1
  Enabled Subsystem/3(Out3) -> Out4/1
  Enabled Subsystem/2(Out2) -> Out3/1
  Enabled Subsystem/1(Out1) -> Out2/1
  S-Function/3 -> Enabled Subsystem/2(In2)
  S-Function/2 -> Enabled Subsystem/1(In1)
  S-Function/1 -> Out1/1, Enabled Subsystem/Enable
  In1/1 -> S-Function/1

== system HANcoder_E407_TTA_CombineModel_Membership_2022a/HANcoder STM32 Target - E407-STM32 algorithm/Message selector/TRLS_ID4_TX/CAN send1 ==
  In1 : Inport
  In2 : Inport  Port=2
  In3 : Inport  Port=3
  In4 : Inport  Port=4
  In5 : Inport  Port=5
  In6 : Inport  Port=6
  In7 : Inport  Port=7
  Gnd8 : Ground
  Gnd9 : Ground
  S-Function : M-S-Function  FunctionName=sfcn_can_send  Parameters=tsamp, canBus, frameType, inputNumber, dataType, byteOrder
  wires:
  In1/1 -> S-Function/1
  In2/1 -> S-Function/2
  In3/1 -> S-Function/3
  In4/1 -> S-Function/4
  In5/1 -> S-Function/5
  In6/1 -> S-Function/6
  In7/1 -> S-Function/7
  Gnd8/1 -> S-Function/8
  Gnd9/1 -> S-Function/9

== system HANcoder_E407_TTA_CombineModel_Membership_2022a/HANcoder STM32 Target - E407-STM32 algorithm/Message selector/TRLS_ID4_TX/uint16to2uint1 ==
  input : Inport
  Bit Shift : hdlsllib/Logic and Bit Operations/Bit Shift  mode=Shift Right Logical  N=8
  Cast : DataTypeConversion  OutDataTypeStr=uint8  SaturateOnIntegerOverflow=off  RndMeth=Floor
  Cast1 : DataTypeConversion  OutDataTypeStr=uint8  SaturateOnIntegerOverflow=off  RndMeth=Floor
  msb : Outport
  lsb : Outport  Port=2
  wires:
  Bit Shift/1 -> Cast/1
  input/1 -> Cast1/1, Bit Shift/1
  Cast/1 -> msb/1
  Cast1/1 -> lsb/1

== system HANcoder_E407_TTA_CombineModel_Membership_2022a/HANcoder STM32 Target - E407-STM32 algorithm/Message selector/TRLS_ID4_TX/uint16to2uint8 ==
  input : Inport
  Bit Shift : hdlsllib/Logic and Bit Operations/Bit Shift  mode=Shift Right Logical  N=8
  Cast : DataTypeConversion  OutDataTypeStr=uint8  SaturateOnIntegerOverflow=off  RndMeth=Floor
  Cast1 : DataTypeConversion  OutDataTypeStr=uint8  SaturateOnIntegerOverflow=off  RndMeth=Floor
  msb : Outport
  lsb : Outport  Port=2
  wires:
  Bit Shift/1 -> Cast/1
  input/1 -> Cast1/1, Bit Shift/1
  Cast/1 -> msb/1
  Cast1/1 -> lsb/1

== system HANcoder_E407_TTA_CombineModel_Membership_2022a/HANcoder STM32 Target - E407-STM32 algorithm/Message selector/TRLS_ID5_RX/2bytes2uint16 ==
  MSB : Inport
  LSB : Inport  Port=2
  Add : Sum
  Bit Shift : hdlsllib/Logic and Bit Operations/Bit Shift  mode=Shift Left Logical  N=8
  Cast : DataTypeConversion  OutDataTypeStr=uint16  SaturateOnIntegerOverflow=off  RndMeth=Floor
  Cast1 : DataTypeConversion  OutDataTypeStr=uint16  SaturateOnIntegerOverflow=off  RndMeth=Floor
  uint16Out : Outport
  wires:
  Cast/1 -> Bit Shift/1
  Bit Shift/1 -> Add/1
  Cast1/1 -> Add/2
  LSB/1 -> Cast1/1
  MSB/1 -> Cast/1
  Add/1 -> uint16Out/1

== system HANcoder_E407_TTA_CombineModel_Membership_2022a/HANcoder STM32 Target - E407-STM32 algorithm/Message selector/TRLS_ID5_RX/CAN receive1 ==
  In1 : Inport
  Enabled Subsystem : Subsystem  TreatAsAtomicUnit=on
  S-Function : M-S-Function  FunctionName=sfcn_can_receive  Parameters=tsamp, canBus, outputNumber, dataType, byteOrder
  Out1 : Outport
  Out2 : Outport  Port=2
  Out3 : Outport  Port=3
  Out4 : Outport  Port=4
  Out5 : Outport  Port=5
  Out6 : Outport  Port=6
  Out7 : Outport  Port=7
  Out8 : Outport  Port=8
  Out9 : Outport  Port=9
  wires:
  S-Function/9 -> Enabled Subsystem/8(In8)
  S-Function/4 -> Enabled Subsystem/3(In3)
  S-Function/5 -> Enabled Subsystem/4(In4)
  S-Function/8 -> Enabled Subsystem/7(In7)
  S-Function/7 -> Enabled Subsystem/6(In6)
  S-Function/6 -> Enabled Subsystem/5(In5)
  Enabled Subsystem/8(Out8) -> Out9/1
  Enabled Subsystem/7(Out7) -> Out8/1
  Enabled Subsystem/6(Out6) -> Out7/1
  Enabled Subsystem/5(Out5) -> Out6/1
  Enabled Subsystem/4(Out4) -> Out5/1
  Enabled Subsystem/3(Out3) -> Out4/1
  Enabled Subsystem/2(Out2) -> Out3/1
  Enabled Subsystem/1(Out1) -> Out2/1
  S-Function/3 -> Enabled Subsystem/2(In2)
  S-Function/2 -> Enabled Subsystem/1(In1)
  S-Function/1 -> Out1/1, Enabled Subsystem/Enable
  In1/1 -> S-Function/1

== system HANcoder_E407_TTA_CombineModel_Membership_2022a/HANcoder STM32 Target - E407-STM32 algorithm/Message selector/TRLS_ID5_TX/CAN send1 ==
  In1 : Inport
  In2 : Inport  Port=2
  In3 : Inport  Port=3
  In4 : Inport  Port=4
  In5 : Inport  Port=5
  In6 : Inport  Port=6
  In7 : Inport  Port=7
  Gnd8 : Ground
  Gnd9 : Ground
  S-Function : M-S-Function  FunctionName=sfcn_can_send  Parameters=tsamp, canBus, frameType, inputNumber, dataType, byteOrder
  wires:
  In1/1 -> S-Function/1
  In2/1 -> S-Function/2
  In3/1 -> S-Function/3
  In4/1 -> S-Function/4
  In5/1 -> S-Function/5
  In6/1 -> S-Function/6
  In7/1 -> S-Function/7
  Gnd8/1 -> S-Function/8
  Gnd9/1 -> S-Function/9

== system HANcoder_E407_TTA_CombineModel_Membership_2022a/HANcoder STM32 Target - E407-STM32 algorithm/Message selector/TRLS_ID5_TX/uint16to2uint1 ==
  input : Inport
  Bit Shift : hdlsllib/Logic and Bit Operations/Bit Shift  mode=Shift Right Logical  N=8
  Cast : DataTypeConversion  OutDataTypeStr=uint8  SaturateOnIntegerOverflow=off  RndMeth=Floor
  Cast1 : DataTypeConversion  OutDataTypeStr=uint8  SaturateOnIntegerOverflow=off  RndMeth=Floor
  msb : Outport
  lsb : Outport  Port=2
  wires:
  Bit Shift/1 -> Cast/1
  input/1 -> Cast1/1, Bit Shift/1
  Cast/1 -> msb/1
  Cast1/1 -> lsb/1

== system HANcoder_E407_TTA_CombineModel_Membership_2022a/HANcoder STM32 Target - E407-STM32 algorithm/Message selector/TRLS_ID5_TX/uint16to2uint2 ==
  input : Inport
  Bit Shift : hdlsllib/Logic and Bit Operations/Bit Shift  mode=Shift Right Logical  N=8
  Cast : DataTypeConversion  OutDataTypeStr=uint8  SaturateOnIntegerOverflow=off  RndMeth=Floor
  Cast1 : DataTypeConversion  OutDataTypeStr=uint8  SaturateOnIntegerOverflow=off  RndMeth=Floor
  msb : Outport
  lsb : Outport  Port=2
  wires:
  Bit Shift/1 -> Cast/1
  Cast/1 -> msb/1
  Cast1/1 -> lsb/1
  input/1 -> Cast1/1, Bit Shift/1

== system HANcoder_E407_TTA_CombineModel_Membership_2022a/HANcoder STM32 Target - E407-STM32 algorithm/Role assignment/Subsystem2/CAN receive1 ==
  In1 : Inport
  Enabled Subsystem : Subsystem  TreatAsAtomicUnit=on
  S-Function : M-S-Function  FunctionName=sfcn_can_receive  Parameters=tsamp, canBus, outputNumber, dataType, byteOrder
  Out1 : Outport
  Out2 : Outport  Port=2
  Out3 : Outport  Port=3
  Out4 : Outport  Port=4
  Out5 : Outport  Port=5
  Out6 : Outport  Port=6
  Out7 : Outport  Port=7
  Out8 : Outport  Port=8
  Out9 : Outport  Port=9
  wires:
  S-Function/9 -> Enabled Subsystem/8(In8)
  S-Function/4 -> Enabled Subsystem/3(In3)
  S-Function/5 -> Enabled Subsystem/4(In4)
  S-Function/8 -> Enabled Subsystem/7(In7)
  S-Function/7 -> Enabled Subsystem/6(In6)
  S-Function/6 -> Enabled Subsystem/5(In5)
  Enabled Subsystem/8(Out8) -> Out9/1
  Enabled Subsystem/7(Out7) -> Out8/1
  Enabled Subsystem/6(Out6) -> Out7/1
  Enabled Subsystem/5(Out5) -> Out6/1
  Enabled Subsystem/4(Out4) -> Out5/1
  Enabled Subsystem/3(Out3) -> Out4/1
  Enabled Subsystem/2(Out2) -> Out3/1
  Enabled Subsystem/1(Out1) -> Out2/1
  S-Function/3 -> Enabled Subsystem/2(In2)
  S-Function/2 -> Enabled Subsystem/1(In1)
  S-Function/1 -> Out1/1, Enabled Subsystem/Enable
  In1/1 -> S-Function/1

== system HANcoder_E407_TTA_CombineModel_Membership_2022a/HANcoder STM32 Target - E407-STM32 algorithm/Role assignment/Subsystem2/Subsystem1 ==
  dataArx : Inport
  Trigger : TriggerPort  VariantControl=(inherit)  PortDimensions=1
  Constant : Constant  Value=0  OutDataTypeStr=uint8
  Constant1 : Constant  OutDataTypeStr=boolean
  Constant2 : Constant  OutDataTypeStr=uint8
  Data Store Write : DataStoreWrite  DataStoreName=SlotTime  IndexOptions=Index vector (dialog)  Indices=1  OutputSizes=1
  Data Store Write1 : DataStoreWrite  DataStoreName=Local_Ticks  IndexOptions=Index vector (dialog)  Indices=1  OutputSizes=1
  Data Store Write2 : DataStoreWrite  DataStoreName=slaveClockOn  IndexOptions=Index vector (dialog)  Indices=1  OutputSizes=1
  Data Store Write3 : DataStoreWrite  DataStoreName=slot  IndexOptions=Index vector (dialog)  Indices=1  OutputSizes=1
  wires:
  dataArx/1 -> Data Store Write/1
  Constant/1 -> Data Store Write1/1
  Constant1/1 -> Data Store Write2/1
  Constant2/1 -> Data Store Write3/1

== system HANcoder_E407_TTA_CombineModel_Membership_2022a/HANcoder STM32 Target - E407-STM32 algorithm/Triggered Subsystem/Subsystem/If Action Subsystem ==
  In1 : Inport
  Action Port : ActionPort
  Out1 : Outport
  wires:
  In1/1 -> Out1/1

== system HANcoder_E407_TTA_CombineModel_Membership_2022a/HANcoder STM32 Target - E407-STM32 algorithm/Triggered Subsystem/Subsystem/If Action Subsystem1 ==
  In1 : Inport
  Action Port : ActionPort
  Gain : Gain  Gain=2
  2 : Outport
  wires:
  In1/1 -> Gain/1
  Gain/1 -> 2/1

== system HANcoder_E407_TTA_CombineModel_Membership_2022a/HANcoder STM32 Target - E407-STM32 algorithm/Triggered Subsystem/Subsystem/If Action Subsystem2 ==
  In1 : Inport
  Action Port : ActionPort
  Out1 : Outport
  wires:
  In1/1 -> Out1/1

== system HANcoder_E407_TTA_CombineModel_Membership_2022a/HANcoder STM32 Target - E407-STM32 algorithm/Triggered Subsystem/Subsystem/If Action Subsystem3 ==
  In1 : Inport
  Action Port : ActionPort
  Gain : Gain  Gain=2
  2 : Outport
  wires:
  In1/1 -> Gain/1
  Gain/1 -> 2/1

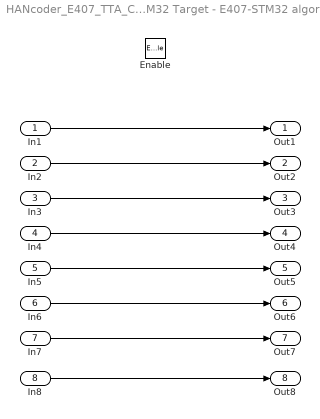
== system HANcoder_E407_TTA_CombineModel_Membership_2022a/HANcoder STM32 Target - E407-STM32 algorithm/Message selector/MMBS1_RX/CAN receive1/Enabled Subsystem ==
  In1 : Inport
  In2 : Inport  Port=2
  In3 : Inport  Port=3
  In4 : Inport  Port=4
  In5 : Inport  Port=5
  In6 : Inport  Port=6
  In7 : Inport  Port=7
  In8 : Inport  Port=8
  Enable : EnablePort
  Out1 : Outport
  Out2 : Outport  Port=2
  Out3 : Outport  Port=3
  Out4 : Outport  Port=4
  Out5 : Outport  Port=5
  Out6 : Outport  Port=6
  Out7 : Outport  Port=7
  Out8 : Outport  Port=8
  wires:
  In8/1 -> Out8/1
  In7/1 -> Out7/1
  In6/1 -> Out6/1
  In5/1 -> Out5/1
  In4/1 -> Out4/1
  In3/1 -> Out3/1
  In2/1 -> Out2/1
  In1/1 -> Out1/1

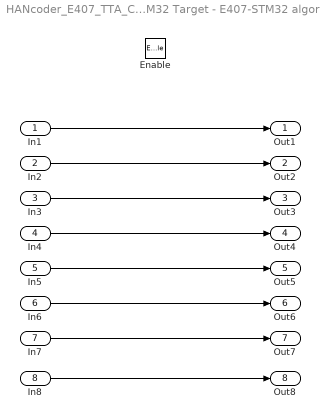
== system HANcoder_E407_TTA_CombineModel_Membership_2022a/HANcoder STM32 Target - E407-STM32 algorithm/Message selector/SSTM1_RX/CAN receive1/Enabled Subsystem ==
  In1 : Inport
  In2 : Inport  Port=2
  In3 : Inport  Port=3
  In4 : Inport  Port=4
  In5 : Inport  Port=5
  In6 : Inport  Port=6
  In7 : Inport  Port=7
  In8 : Inport  Port=8
  Enable : EnablePort
  Out1 : Outport
  Out2 : Outport  Port=2
  Out3 : Outport  Port=3
  Out4 : Outport  Port=4
  Out5 : Outport  Port=5
  Out6 : Outport  Port=6
  Out7 : Outport  Port=7
  Out8 : Outport  Port=8
  wires:
  In8/1 -> Out8/1
  In7/1 -> Out7/1
  In6/1 -> Out6/1
  In5/1 -> Out5/1
  In4/1 -> Out4/1
  In3/1 -> Out3/1
  In2/1 -> Out2/1
  In1/1 -> Out1/1

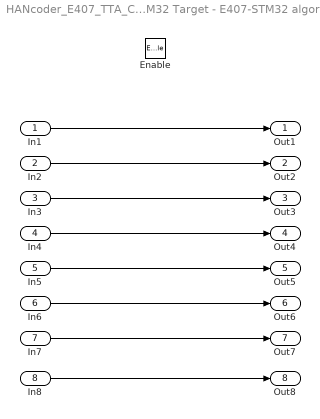
== system HANcoder_E407_TTA_CombineModel_Membership_2022a/HANcoder STM32 Target - E407-STM32 algorithm/Message selector/SYNC1_RX/CAN receive1/Enabled Subsystem ==
  In1 : Inport
  In2 : Inport  Port=2
  In3 : Inport  Port=3
  In4 : Inport  Port=4
  In5 : Inport  Port=5
  In6 : Inport  Port=6
  In7 : Inport  Port=7
  In8 : Inport  Port=8
  Enable : EnablePort
  Out1 : Outport
  Out2 : Outport  Port=2
  Out3 : Outport  Port=3
  Out4 : Outport  Port=4
  Out5 : Outport  Port=5
  Out6 : Outport  Port=6
  Out7 : Outport  Port=7
  Out8 : Outport  Port=8
  wires:
  In8/1 -> Out8/1
  In7/1 -> Out7/1
  In6/1 -> Out6/1
  In5/1 -> Out5/1
  In4/1 -> Out4/1
  In3/1 -> Out3/1
  In2/1 -> Out2/1
  In1/1 -> Out1/1

== system HANcoder_E407_TTA_CombineModel_Membership_2022a/HANcoder STM32 Target - E407-STM32 algorithm/Message selector/Slot 5 execution/Inputs/Quadrature Encoder Get ==
  Data Type Conversion : DataTypeConversion  OutDataTypeStr=boolean  SaturateOnIntegerOverflow=off  RndMeth=Floor
  Detect Increase : simulink/Logic and Bit Operations/Detect Increase  vinit=0.0  OutDataTypeStr=uint8
  Gnd1 : Ground
  Level-2 M-file S-Function : M-S-Function  FunctionName=sfcn_quad_encoder_get  Parameters=tsamp, moduleID
  Out1 : Outport
  wires:
  Level-2 M-file S-Function/1 -> Out1/1
  Gnd1/1 -> Detect Increase/1
  Detect Increase/1 -> Data Type Conversion/1
  Data Type Conversion/1 -> Level-2 M-file S-Function/1

== system HANcoder_E407_TTA_CombineModel_Membership_2022a/HANcoder STM32 Target - E407-STM32 algorithm/Message selector/Slot 5 execution/Outputs/PWM Init ==
  S-Function : S-Function  FunctionName=sfcn_pwmout_init  SFunctionDeploymentMode=off  EnableBusSupport=off
  Term1 : Terminator
  wires:
  S-Function/1 -> Term1/1

== system HANcoder_E407_TTA_CombineModel_Membership_2022a/HANcoder STM32 Target - E407-STM32 algorithm/Message selector/Subsystem/Kinematic Algorithm/1st trailer local velocity ==
  Gamma2 : Inport
  V2 : Inport  Port=2
  L1F : Inport  Port=3
  ThetaDot2 : Inport  Port=4
  Add : Sum
  Cast : DataTypeConversion  SaturateOnIntegerOverflow=off  RndMeth=Floor
  Product1 : Product  Inputs=**
  Product2 : Product  Inputs=***
  tan 1 : Trigonometry
  tan 2 : Trigonometry  Operator=cos
  V1 : Outport
  wires:
  tan 1/1 -> Product2/3
  tan 2/1 -> Product1/1
  Gamma2/1 -> Cast/1
  L1F/1 -> Product2/2
  V2/1 -> Product1/2
  Product2/1 -> Add/1  "L1f * ThetaDot2*sin(gamma2)"
  Product1/1 -> Add/2  "v2*cos(gamma2)"
  Add/1 -> V1/1
  ThetaDot2/1 -> Product2/1
  Cast/1 -> tan 1/1, tan 2/1
